simulink model "Mdl_Examle02"  (Simulink 6.1)
settings: Solver=ode4  StartTime=0.0  StopTime=2  FixedStep=0.01  RelTol=1e-3
values from neighbouring files (symbols this model uses):
  A = [1 0 0;3 -1 1;0 2 0]    [Example02.m]
  B = [2 1 1]'    [Example02.m]
  C = [0 0 1]    [Example02.m]
  G = K_couple'    [Example02.m]
settings Model: LastModifiedBy=ybstrong
settings DebuggingCC: SolverPrmCheckMsg=warning

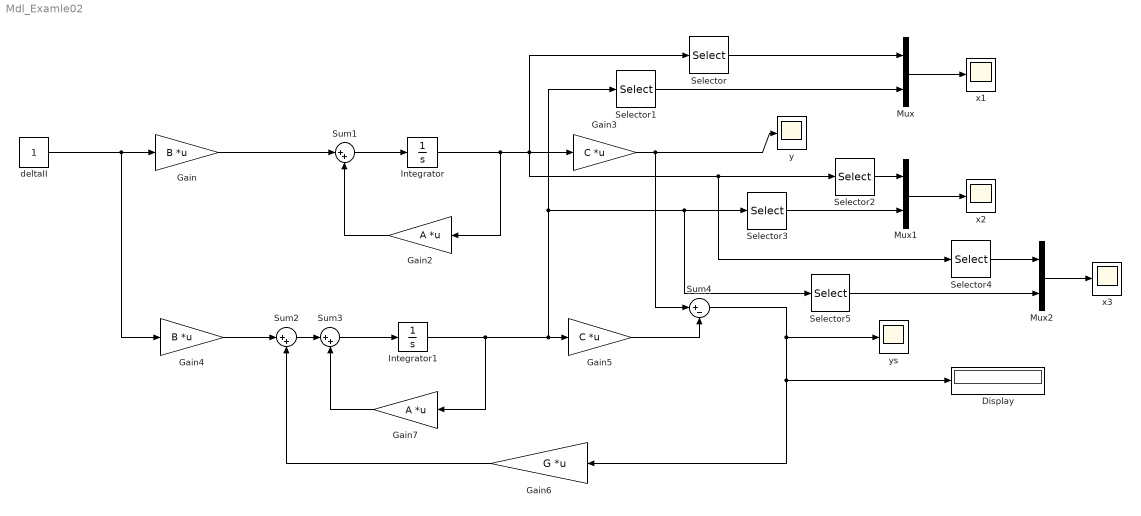
== system Mdl_Examle02 ==
  Display : Display
  Gain : Gain  Gain=B  Multiplication=Matrix(K*u)
  Gain2 : Gain  Orientation=left  Gain=A  Multiplication=Matrix(K*u)
  Gain3 : Gain  Gain=C  Multiplication=Matrix(K*u)
  Gain4 : Gain  Gain=B  Multiplication=Matrix(K*u)
  Gain5 : Gain  Gain=C  Multiplication=Matrix(K*u)
  Gain6 : Gain  Orientation=left  Gain=G  Multiplication=Matrix(K*u)
  Gain7 : Gain  Orientation=left  Gain=A  Multiplication=Matrix(K*u)
  Integrator : Integrator  InitialCondition=[0;1;2]
  Integrator1 : Integrator
  Mux : Mux  Inputs=2
  Mux1 : Mux  Inputs=2
  Mux2 : Mux  Inputs=2
  Selector : Selector  InputPortWidth=3
  Selector1 : Selector  InputPortWidth=3
  Selector2 : Selector  Elements=2  InputPortWidth=3
  Selector3 : Selector  Elements=2  InputPortWidth=3
  Selector4 : Selector  Elements=3  InputPortWidth=3
  Selector5 : Selector  Elements=3  InputPortWidth=3
  Sum1 : Sum  Inputs=|++
  Sum2 : Sum  Inputs=|++
  Sum3 : Sum  Inputs=|++
  Sum4 : Sum  Inputs=|+-
  deltaII : Constant
  x1 : Scope
  x2 : Scope
      settings: SaveName=ScopeData3
  x3 : Scope
      settings: SaveName=ScopeData4
  y : Scope
  ys : Scope
      settings: SaveName=ScopeData2
  wires:
  deltaII/1 -> Gain/1, Gain4/1
  Gain/1 -> Sum1/1
  Sum1/1 -> Integrator/1
  Integrator/1 -> Gain2/1, Gain3/1, Selector/1, Selector2/1, Selector4/1
  Gain2/1 -> Sum1/2
  Gain3/1 -> Sum4/1, y/1
  Gain4/1 -> Sum2/1
  Sum2/1 -> Sum3/1
  Integrator1/1 -> Gain7/1, Gain5/1, Selector1/1, Selector3/1, Selector5/1
  Sum3/1 -> Integrator1/1
  Gain5/1 -> Sum4/2
  Sum4/1 -> ys/1, Gain6/1, Display/1
  Gain6/1 -> Sum2/2
  Gain7/1 -> Sum3/2
  Mux/1 -> x1/1
  Selector/1 -> Mux/1
  Selector1/1 -> Mux/2
  Selector2/1 -> Mux1/1
  Selector3/1 -> Mux1/2
  Mux1/1 -> x2/1
  Selector4/1 -> Mux2/1
  Selector5/1 -> Mux2/2
  Mux2/1 -> x3/1
